simulink model "Demo1"  (R2018b)
settings: Solver=FixedStepDiscrete  StartTime=0.0  StopTime=10  FixedStep=0.0005  RelTol=1e-3  EnableMultiTasking=on
undefined symbols (not defined in the file or in its folder): ADS1, ADS2, br_opening, BRAKE, I_AN06_5V, I_AN08_5V, I_AN09_5V, I_AN10_5V, I_HALL1, I_HALL2, I_SW11_H, I_SW16_H, MnPedal_H, MnPedal_L, MxPedal_H, MxPedal_L, O_PWM1_LS0A7, O_PWM2_LS0A7, O_SW02_LS0A4, O_SW13_HS1A, O_SW14_HS1A, PUMP, th_opening
libraries: ec5744lib x93, canmsglib x14, simulink x5
(part 1 of 2)
settings Model: Creator=30855  LastModifiedBy=30855
settings OptimizationCC: DefaultParameterBehavior=Inlined  InlineInvariantSignals=on  EnhancedBackFolding=on  ExpressionFolding=off  PassReuseOutputArgsAs=Individual arguments  RollThreshold=65  StateBitsets=on  DataBitsets=on  ZeroExternalMemoryAtStartup=off  ZeroInternalMemoryAtStartup=off  EfficientFloat2IntCast=on  OptimizeBlockOrder=speed  DifferentSizesBufferReuse=on
settings DebuggingCC: InheritedTsInSrcMsg=none  ParameterTunabilityLossMsg=error
settings HardwareCC: ProdBitPerPointer=32  ProdBitPerSizeT=32  ProdBitPerPtrDiffT=32  ProdLargestAtomicInteger=Long  ProdLargestAtomicFloat=Double  ProdEndianess=BigEndian  ProdWordSize=32  ProdHWDeviceType=Freescale MPC5500
settings SFSimCC: MATLABDynamicMemAlloc=off
settings RTWCC: SystemTargetFile=ec5744.tlc  MakeCommand=make_rtw optimized_fixed_point=1  GenerateMakefile=off  TemplateMakefile=ec5744_lcc.tmf  PostCodeGenCommand=ec5744_pst_s2(buildInfo)  Description=Target for EC5744  GenerateReport=on  IncludeHyperlinkInReport=on  LaunchReport=on  GenerateTraceInfo=on  GenerateTraceReport=on  GenerateTraceReportSl=on  GenerateTraceReportSf=on  GenerateTraceReportEml=on
settings CodeAppCC: ForceParamTrailComments=on  IgnoreCustomStorageClasses=off  OperatorAnnotations=on  SimulinkDataObjDesc=on  SFDataObjDesc=on  InsertBlockDesc=on
settings STFCustomTargetCC: TargetLangStandard=C99 (ISO)  MultiwordLength=256  ModelReferenceCompliant=off  IncludeMdlTerminateFcn=off  CombineOutputUpdateFcns=on  SuppressErrorStatus=on  ERTCustomFileBanners=on  SupportContinuousTime=off  SupportNonInlinedSFcns=off  RemoveResetFunc=on  MATLABClassNameForMDSCustomization=Simulink.SoftwareTarget.ERTCustomization  SystemTargetFile=ec5744.tlc
settings ERTTargetCC: TargetLangStandard=C99 (ISO)  ModelReferenceCompliant=off  ParMdlRefBuildCompliant=off  CompOptLevelCompliant=off  ConcurrentExecutionCompliant=off  IncludeMdlTerminateFcn=off  SuppressErrorStatus=on  ModelStepFunctionPrototypeControlCompliant=off  CPPClassGenCompliant=off  UseToolchainInfoCompliant=off  GenerateASAP2=on  InlinedParameterPlacement=NonHierarchical  ERTSrcFileBannerTemplate=ec5744_code_template.cgt  ERTHdrFileBannerTemplate=ec5744_code_template.cgt  ERTDataSrcFileTemplate=ec5744_code_template.cgt  ERTDataHdrFileTemplate=ec5744_code_template.cgt  ERTCustomFileTemplate=ec5744_file_process.tlc

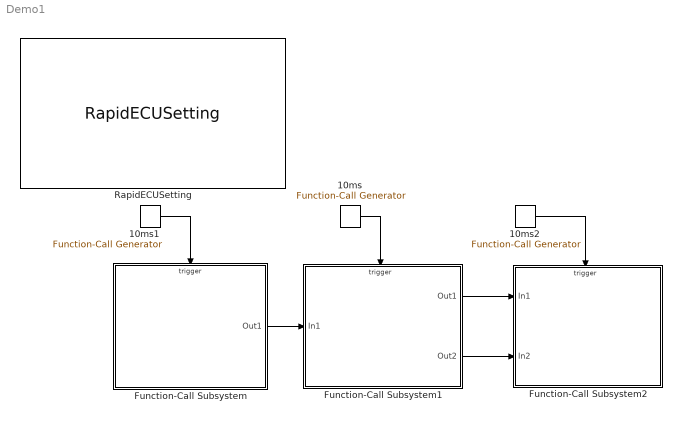
== system Demo1 ==
  10ms : simulink/Ports & Subsystems/Function-Call Generator  sample_time=0.01  numberOfIterations=1
  10ms1 : simulink/Ports & Subsystems/Function-Call Generator  sample_time=0.01  numberOfIterations=1
  10ms2 : simulink/Ports & Subsystems/Function-Call Generator  sample_time=0.01  numberOfIterations=1
  Function-Call Subsystem : Subsystem  TreatAsAtomicUnit=on
  Function-Call Subsystem1 : Subsystem  TreatAsAtomicUnit=on
  Function-Call Subsystem2 : Subsystem  TreatAsAtomicUnit=on
  RapidECUSetting : ec5744lib/RapidECU_U3/RapidECUSetting
      link override CAN: apdf=9  acmt=Extended(29-bit ID)  bpdf=9  cpdf=9  aboi=off  bcmt=Extended(29-bit ID)
      link override LIN: abrt=19200
      settings: SourceProductName=ECUCoder for MPC5744
  wires:
  10ms/1 -> Function-Call Subsystem1/Trigger
  Function-Call Subsystem/1(Out1) -> Function-Call Subsystem1/1(In1)
  Function-Call Subsystem1/1(Out1) -> Function-Call Subsystem2/1(In1)
  Function-Call Subsystem1/2(Out2) -> Function-Call Subsystem2/2(In2)
  10ms1/1 -> Function-Call Subsystem/Trigger
  10ms2/1 -> Function-Call Subsystem2/Trigger

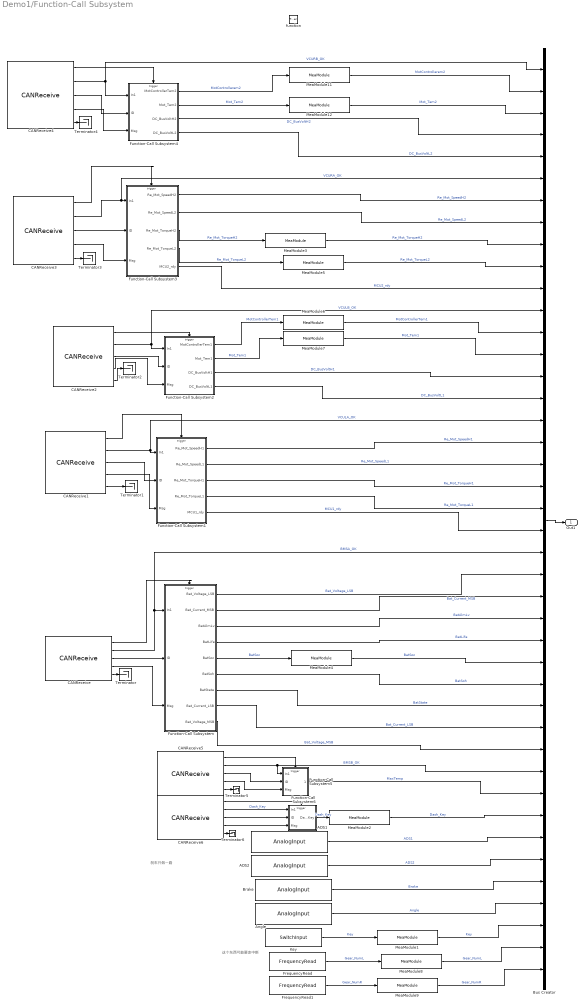
== system Demo1/Function-Call Subsystem ==
  note: 这个东西可能要走中断
  note: 刹车只做一路
  function : TriggerPort  TriggerType=function-call  VariantControl=Variant
  ADS1 : ec5744lib/RapidECU_U3/01BasicInput/AnalogInput  channel=54:I_AN08_5V  sampletime=-1
      settings: SourceProductName=ECUCoder for MPC5744
  ADS2 : ec5744lib/RapidECU_U3/01BasicInput/AnalogInput  channel=55:I_AN09_5V  sampletime=-1
      settings: SourceProductName=ECUCoder for MPC5744
  Angle : ec5744lib/RapidECU_U3/01BasicInput/AnalogInput  channel=56:I_AN10_5V  sampletime=-1
      settings: SourceProductName=ECUCoder for MPC5744
  Brake : ec5744lib/RapidECU_U3/01BasicInput/AnalogInput  channel=52:I_AN06_5V  sampletime=-1
      settings: SourceProductName=ECUCoder for MPC5744
  Bus Creator : BusCreator  Inputs=42
  CANReceive : ec5744lib/RapidECU_U3/04CANCommunication/CANReceive  canmodule=0  canbuffer=1  canmessageid=hex2dec('186040F3')  canmessagetype=Extended(29-bit ID)  datalength=8  sampletime=-1
      settings: SourceProductName=ECUCoder for MPC5744
  CANReceive1 : ec5744lib/RapidECU_U3/04CANCommunication/CANReceive  canmodule=1  canbuffer=6  canmessageid=hex2dec('CFFC6EF')  canmessagetype=Extended(29-bit ID)  datalength=8  sampletime=-1
      settings: SourceProductName=ECUCoder for MPC5744
  CANReceive2 : ec5744lib/RapidECU_U3/04CANCommunication/CANReceive  canmodule=1  canbuffer=4  canmessageid=hex2dec('CFFC7EF')  canmessagetype=Extended(29-bit ID)  datalength=8  sampletime=-1
      settings: SourceProductName=ECUCoder for MPC5744
  CANReceive3 : ec5744lib/RapidECU_U3/04CANCommunication/CANReceive  canmodule=1  canbuffer=2  canmessageid=hex2dec('CB221EF')  canmessagetype=Extended(29-bit ID)  datalength=8  sampletime=-1
      settings: SourceProductName=ECUCoder for MPC5744
  CANReceive4 : ec5744lib/RapidECU_U3/04CANCommunication/CANReceive  canmodule=1  canbuffer=0  canmessageid=hex2dec('CB321EF')  canmessagetype=Extended(29-bit ID)  datalength=8  sampletime=-1
      settings: SourceProductName=ECUCoder for MPC5744
  CANReceive5 : ec5744lib/RapidECU_U3/04CANCommunication/CANReceive  canmodule=0  canbuffer=3  canmessageid=hex2dec('186240F3')  canmessagetype=Extended(29-bit ID)  datalength=8  sampletime=-1
      settings: SourceProductName=ECUCoder for MPC5744
  CANReceive6 : ec5744lib/RapidECU_U3/04CANCommunication/CANReceive  canmodule=0  canbuffer=5  canmessageid=hex2dec('155')  canmessagetype=Extended(29-bit ID)  datalength=8  sampletime=-1
      settings: SourceProductName=ECUCoder for MPC5744
  FrequencyRead : ec5744lib/RapidECU_U3/01BasicInput/FrequencyRead  channel=37:I_HALL1  sampletime=-1
      settings: SourceProductName=ECUCoder for MPC5744
  FrequencyRead1 : ec5744lib/RapidECU_U3/01BasicInput/FrequencyRead  channel=103:I_SW16_H/I_HALL2  sampletime=-1
      settings: SourceProductName=ECUCoder for MPC5744
  Function-Call Subsystem : Subsystem  TreatAsAtomicUnit=on
  Function-Call Subsystem1 : Subsystem  TreatAsAtomicUnit=on
  Function-Call Subsystem2 : Subsystem  TreatAsAtomicUnit=on
  Function-Call Subsystem3 : Subsystem  TreatAsAtomicUnit=on
  Function-Call Subsystem4 : Subsystem  TreatAsAtomicUnit=on
  Function-Call Subsystem5 : Subsystem  TreatAsAtomicUnit=on
  Function-Call Subsystem6 : Subsystem  TreatAsAtomicUnit=on
  Key : ec5744lib/RapidECU_U3/01BasicInput/SwitchInput  channel=44:I_SW11_H  sampletime=-1
      settings: SourceProductName=ECUCoder for MPC5744
  MeaModule1 : ec5744lib/RapidECU_U3/07Calibration/MeaModule  signal=Key
      settings: SourceProductName=ECUCoder for MPC5744
  MeaModule11 : ec5744lib/RapidECU_U3/07Calibration/MeaModule  signal=MotConTem2
      settings: SourceProductName=ECUCoder for MPC5744
  MeaModule12 : ec5744lib/RapidECU_U3/07Calibration/MeaModule  signal=MotTem2
      settings: SourceProductName=ECUCoder for MPC5744
  MeaModule2 : ec5744lib/RapidECU_U3/07Calibration/MeaModule  signal=Dash_Key
      settings: SourceProductName=ECUCoder for MPC5744
  MeaModule3 : ec5744lib/RapidECU_U3/07Calibration/MeaModule  signal=Re_Mot_ToqH
      settings: SourceProductName=ECUCoder for MPC5744
  MeaModule4 : ec5744lib/RapidECU_U3/07Calibration/MeaModule  signal=BatSoc
      settings: SourceProductName=ECUCoder for MPC5744
  MeaModule5 : ec5744lib/RapidECU_U3/07Calibration/MeaModule  signal=Re_MotToqL
      settings: SourceProductName=ECUCoder for MPC5744
  MeaModule6 : ec5744lib/RapidECU_U3/07Calibration/MeaModule  signal=MotConTem1
      settings: SourceProductName=ECUCoder for MPC5744
  MeaModule7 : ec5744lib/RapidECU_U3/07Calibration/MeaModule  signal=MotTem1
      settings: SourceProductName=ECUCoder for MPC5744
  MeaModule8 : ec5744lib/RapidECU_U3/07Calibration/MeaModule  signal=HTime_L
      settings: SourceProductName=ECUCoder for MPC5744
  MeaModule9 : ec5744lib/RapidECU_U3/07Calibration/MeaModule  signal=HTime_R
      settings: SourceProductName=ECUCoder for MPC5744
  Terminator{,1..6} (7 alike) : Terminator
  Out1 : Outport
  wires:
  ADS1/1 -> Bus Creator/36  "ADS1"
  ADS2/1 -> Bus Creator/37  "ADS2"
  Brake/1 -> Bus Creator/38  "Brake"
  Angle/1 -> Bus Creator/39  "Angle"
  Bus Creator/1 -> Out1/1
  Key/1 -> MeaModule1/1  "Key"
  CANReceive/1 -> Function-Call Subsystem/Trigger
  CANReceive/2 -> Bus Creator/23, Function-Call Subsystem/1(In1)  "BMSA_OK"
  CANReceive/3 -> Function-Call Subsystem/2(ID)
  CANReceive/4 -> Function-Call Subsystem/3(Msg)
  CANReceive/5 -> Terminator/1
  Function-Call Subsystem/1(Bat_Voltage_LSB) -> Bus Creator/24  "Bat_Voltage_LSB"
  Function-Call Subsystem/2(Bat_Current_MSB) -> Bus Creator/25  "Bat_Current_MSB"
  Function-Call Subsystem/3(BatAlmLv) -> Bus Creator/26  "BatAlmLv"
  Function-Call Subsystem/4(BatLife) -> Bus Creator/27  "BatLife"
  Function-Call Subsystem/5(BatSoc) -> MeaModule4/1  "BatSoc"
  Function-Call Subsystem/6(BatSoh) -> Bus Creator/29  "BatSoh"
  Function-Call Subsystem/7(BatState) -> Bus Creator/30  "BatState"
  Function-Call Subsystem/8(Bat_Current_LSB) -> Bus Creator/31  "Bat_Current_LSB"
  FrequencyRead/1 -> MeaModule8/1  "Gear_NumL"
  CANReceive1/5 -> Terminator1/1
  CANReceive1/4 -> Function-Call Subsystem1/3(Msg)
  CANReceive1/3 -> Function-Call Subsystem1/2(ID)
  CANReceive1/2 -> Bus Creator/17, Function-Call Subsystem1/1(In1)  "VCULA_OK"
  CANReceive1/1 -> Function-Call Subsystem1/Trigger
  CANReceive2/1 -> Function-Call Subsystem2/Trigger
  CANReceive2/2 -> Function-Call Subsystem2/1(In1), Bus Creator/12  "VCULB_OK"
  CANReceive2/3 -> Function-Call Subsystem2/2(ID)
  CANReceive2/4 -> Function-Call Subsystem2/3(Msg)
  CANReceive2/5 -> Terminator2/1
  CANReceive3/5 -> Terminator3/1
  CANReceive3/4 -> Function-Call Subsystem3/3(Msg)
  CANReceive3/3 -> Function-Call Subsystem3/2(ID)
  CANReceive3/2 -> Bus Creator/6, Function-Call Subsystem3/1(In1)  "VCURA_OK"
  CANReceive3/1 -> Function-Call Subsystem3/Trigger
  CANReceive4/1 -> Function-Call Subsystem4/Trigger
  CANReceive4/2 -> Bus Creator/1, Function-Call Subsystem4/1(In1)  "VCURB_OK"
  CANReceive4/3 -> Function-Call Subsystem4/2(ID)
  CANReceive4/4 -> Function-Call Subsystem4/3(Msg)
  CANReceive4/5 -> Terminator4/1
  Function-Call Subsystem1/4(Re_Mot_TorqueL1) -> Bus Creator/21  "Re_Mot_TorqueL1"
  Function-Call Subsystem1/3(Re_Mot_TorqueH1) -> Bus Creator/20  "Re_Mot_TorqueH1"
  Function-Call Subsystem1/2(Re_Mot_SpeedL1) -> Bus Creator/19  "Re_Mot_SpeedL1"
  Function-Call Subsystem1/1(Re_Mot_SpeedH1) -> Bus Creator/18  "Re_Mot_SpeedH1"
  Function-Call Subsystem2/2(Mot_Tem1) -> MeaModule7/1  "Mot_Tem1"
  Function-Call Subsystem2/1(MotControllerTem1) -> MeaModule6/1  "MotControllerTem1"
  Function-Call Subsystem3/4(Re_Mot_TorqueL2) -> MeaModule5/1  "Re_Mot_TorqueL2"
  Function-Call Subsystem3/3(Re_Mot_TorqueH2) -> MeaModule3/1  "Re_Mot_TorqueH2"
  Function-Call Subsystem3/2(Re_Mot_SpeedL2) -> Bus Creator/8  "Re_Mot_SpeedL2"
  Function-Call Subsystem3/1(Re_Mot_SpeedH2) -> Bus Creator/7  "Re_Mot_SpeedH2"
  Function-Call Subsystem4/2(Mot_Tem2) -> MeaModule12/1  "Mot_Tem2"
  Function-Call Subsystem4/1(MotControllerTem2) -> MeaModule11/1  "MotControllerem2"
  Function-Call Subsystem/9(Bat_Voltage_MSB) -> Bus Creator/32  "Bat_Voltage_MSB"
  CANReceive5/5 -> Terminator5/1
  CANReceive5/4 -> Function-Call Subsystem5/3(Msg)
  CANReceive5/3 -> Function-Call Subsystem5/2(ID)
  CANReceive5/2 -> Bus Creator/33, Function-Call Subsystem5/1(In1)  "BMSB_OK"
  CANReceive5/1 -> Function-Call Subsystem5/Trigger
  Function-Call Subsystem5/1(MaxTemp) -> Bus Creator/34  "MaxTemp"
  FrequencyRead1/1 -> MeaModule9/1  "Gear_NumR"
  CANReceive6/1 -> Function-Call Subsystem6/Trigger
  CANReceive6/3 -> Function-Call Subsystem6/2(ID)
  CANReceive6/4 -> Function-Call Subsystem6/3(Msg)
  CANReceive6/5 -> Terminator6/1
  Function-Call Subsystem6/1(Dash_Key) -> MeaModule2/1  "Dash_Key"
  MeaModule1/1 -> Bus Creator/40  "Key"
  MeaModule3/1 -> Bus Creator/9  "Re_Mot_TorqueH2"
  MeaModule5/1 -> Bus Creator/10  "Re_Mot_TorqueL2"
  MeaModule6/1 -> Bus Creator/13  "MotControllerTem1"
  MeaModule7/1 -> Bus Creator/14  "Mot_Tem1"
  MeaModule8/1 -> Bus Creator/41  "Gear_NumL"
  MeaModule9/1 -> Bus Creator/42  "Gear_NumR"
  MeaModule11/1 -> Bus Creator/2  "MotControllerem2"
  MeaModule12/1 -> Bus Creator/3  "Mot_Tem2"
  MeaModule2/1 -> Bus Creator/35  "Dash_Key"
  CANReceive6/2 -> Function-Call Subsystem6/1(In1)  "Dash_Key"
  Function-Call Subsystem2/3(DC_BusVoltH1) -> Bus Creator/15  "DC_BusVoltH1"
  Function-Call Subsystem4/3(DC_BusVoltH2) -> Bus Creator/4  "DC_BusVoltH2"
  Function-Call Subsystem4/4(DC_BusVoltL2) -> Bus Creator/5  "DC_BusVoltL2"
  Function-Call Subsystem2/4(DC_BusVoltL1) -> Bus Creator/16  "DC_BusVoltL1"
  MeaModule4/1 -> Bus Creator/28  "BatSoc"
  Function-Call Subsystem1/5(MCU1_rdy) -> Bus Creator/22  "MCU1_rdy"
  Function-Call Subsystem3/5(MCU2_rdy) -> Bus Creator/11  "MCU2_rdy"

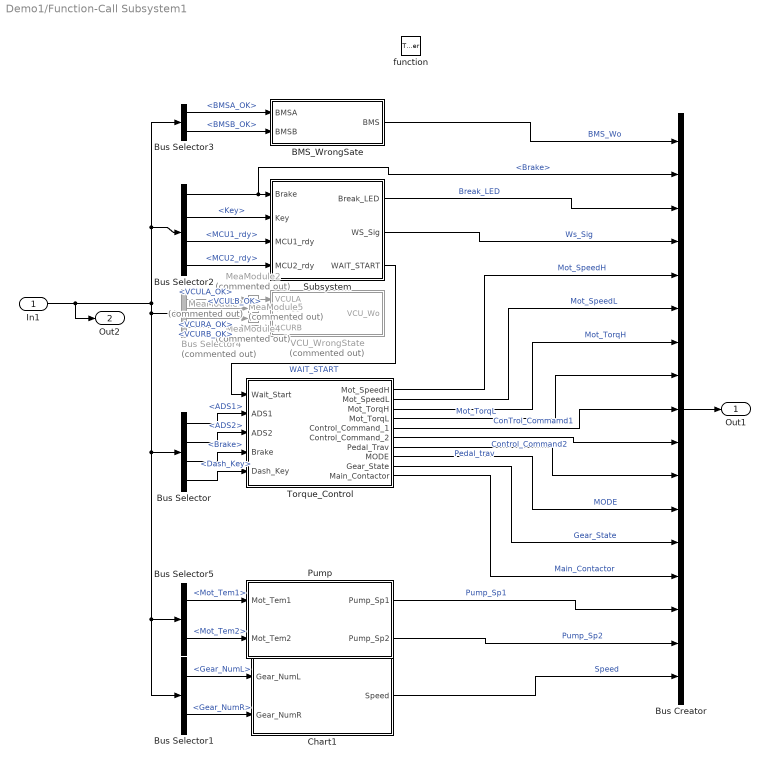
== system Demo1/Function-Call Subsystem1 ==
  In1 : Inport
  "  function" : TriggerPort  TriggerType=function-call  VariantControl=Variant
  BMS_WrongSate : Stateflow chart  TreatAsAtomicUnit=on
  Bus Creator : BusCreator  Inputs=17
  Bus Selector : BusSelector  OutputSignals=ADS1,ADS2,Brake,Dash_Key
  Bus Selector1 : BusSelector  OutputSignals=Gear_NumL,Gear_NumR
  Bus Selector2 : BusSelector  OutputSignals=Brake,Key,MCU1_rdy,MCU2_rdy
  Bus Selector3 : BusSelector  OutputSignals=BMSA_OK,BMSB_OK
  Bus Selector4 : BusSelector  Commented=on  OutputSignals=VCULA_OK,VCULB_OK,VCURA_OK,VCURB_OK
  Bus Selector5 : BusSelector  OutputSignals=Mot_Tem1,Mot_Tem2
  Chart1 : Stateflow chart  TreatAsAtomicUnit=on
  MeaModule2 : ec5744lib/RapidECU_U3/07Calibration/MeaModule  Commented=on  signal=VCULA
      settings: SourceProductName=ECUCoder for MPC5744
  MeaModule3 : ec5744lib/RapidECU_U3/07Calibration/MeaModule  Commented=on  signal=VCUlb
      settings: SourceProductName=ECUCoder for MPC5744
  MeaModule4 : ec5744lib/RapidECU_U3/07Calibration/MeaModule  Commented=on  signal=VCUra
      settings: SourceProductName=ECUCoder for MPC5744
  MeaModule5 : ec5744lib/RapidECU_U3/07Calibration/MeaModule  Commented=on  signal=VCUrb
      settings: SourceProductName=ECUCoder for MPC5744
  Pump : Subsystem
  Subsystem : Subsystem
  Torque_Control : Subsystem
  VCU_WrongState : Stateflow chart  Commented=on  TreatAsAtomicUnit=on
  Out1 : Outport
  Out2 : Outport  Port=2
  wires:
  Bus Selector/1 -> Torque_Control/2(ADS1)  "<ADS1>"
  Bus Selector/2 -> Torque_Control/3(ADS2)  "<ADS2>"
  Torque_Control/1(Mot_SpeedH) -> Bus Creator/5  "Mot_SpeedH"
  Torque_Control/2(Mot_SpeedL) -> Bus Creator/6  "Mot_SpeedL"
  Torque_Control/3(Mot_TorqH) -> Bus Creator/7  "Mot_TorqH"
  Torque_Control/4(Mot_TorqL) -> Bus Creator/8  "Mot_TorqL"
  Bus Creator/1 -> Out1/1
  Bus Selector2/2 -> Subsystem/2(Key)  "<Key>"
  Subsystem/3(WAIT_START) -> Torque_Control/1(Wait_Start)  "WAIT_START"
  BMS_WrongSate/1(BMS) -> Bus Creator/1  "BMS_Wo"
  Torque_Control/5("Control_Command_1 ") -> Bus Creator/9  "ConTrol_Commamd1"
  Torque_Control/6(Control_Command_2) -> Bus Creator/10  "Control_Command2"
  Bus Selector2/1 -> Bus Creator/2, Subsystem/1(Brake)  "<Brake>"
  Torque_Control/7(Pedal_Trav) -> Bus Creator/11  "Pedal_trav"
  Bus Selector/4 -> Torque_Control/5("Dash_Key ")  "<Dash_Key>"
  Bus Selector5/1 -> Pump/1(Mot_Tem1)  "<Mot_Tem1>"
  Bus Selector5/2 -> Pump/2(Mot_Tem2)  "<Mot_Tem2>"
  Pump/1(Pump_Sp1) -> Bus Creator/15  "Pump_Sp1"
  Pump/2(Pump_Sp2) -> Bus Creator/16  "Pump_Sp2"
  Subsystem/1(Break_LED) -> Bus Creator/3  "Break_LED"
  Bus Selector/3 -> Torque_Control/4("Brake ")  "<Brake>"
  Bus Selector3/1 -> BMS_WrongSate/1(BMSA)  "<BMSA_OK>"
  Bus Selector3/2 -> BMS_WrongSate/2(BMSB)  "<BMSB_OK>"
  Bus Selector4/1 -> MeaModule2/1  "<VCULA_OK>"
  Bus Selector4/2 -> MeaModule3/1  "<VCULB_OK>"
  Bus Selector4/3 -> MeaModule4/1  "<VCURA_OK>"
  Bus Selector4/4 -> MeaModule5/1  "<VCURB_OK>"
  MeaModule2/1 -> VCU_WrongState/1(VCULA)
  MeaModule3/1 -> VCU_WrongState/2(VCULB)
  MeaModule4/1 -> VCU_WrongState/3(VCURA)
  MeaModule5/1 -> VCU_WrongState/4(VCURB)
  Bus Selector1/2 -> Chart1/2(Gear_NumR)  "<Gear_NumR>"
  Bus Selector1/1 -> Chart1/1(Gear_NumL)  "<Gear_NumL>"
  In1/1 -> Out2/1, Bus Selector4/1, Bus Selector1/1, Bus Selector5/1, Bus Selector/1, Bus Selector3/1, Bus Selector2/1
  Chart1/1(Speed) -> Bus Creator/17  "Speed"
  Torque_Control/8(MODE) -> Bus Creator/12  "MODE"
  Subsystem/2(WS_Sig) -> Bus Creator/4  "Ws_Sig"
  Torque_Control/9("Gear_State ") -> Bus Creator/13  "Gear_State"
  Torque_Control/10(Main_Contactor) -> Bus Creator/14  "Main_Contactor"
  Bus Selector2/3 -> Subsystem/3(MCU1_rdy)  "<MCU1_rdy>"
  Bus Selector2/4 -> Subsystem/4(MCU2_rdy)  "<MCU2_rdy>"

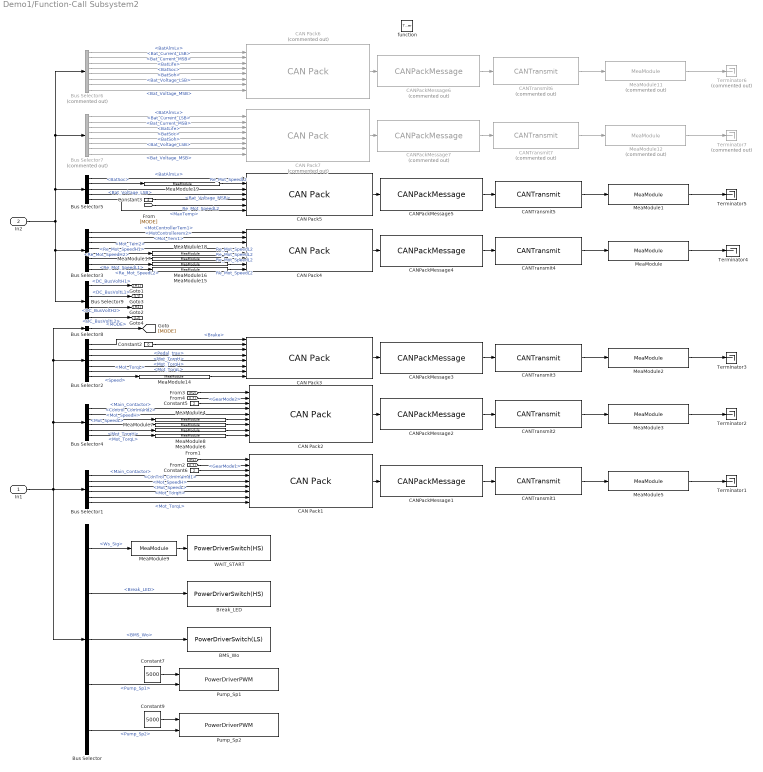
== system Demo1/Function-Call Subsystem2 ==
  In1 : Inport
  In2 : Inport  Port=2
  function : TriggerPort  TriggerType=function-call  VariantControl=Variant
  BMS_Wo : ec5744lib/RapidECU_U3/02PowerDriverSwitch/PowerDriverSwitch(LS)  channel=59:O_SW02_LS0A4  sampletime=-1
      settings: SourceProductName=ECUCoder for MPC5744
  Break_LED : ec5744lib/RapidECU_U3/02PowerDriverSwitch/PowerDriverSwitch(HS)  channel=115:O_SW13_HS1A  sampletime=-1
      settings: SourceProductName=ECUCoder for MPC5744
  Bus Selector : BusSelector  OutputSignals=Ws_Sig,Break_LED,BMS_Wo,Pump_Sp1,Pump_Sp2
  Bus Selector1 : BusSelector  OutputSignals=Main_Contactor,ConTrol_Commamd1,Mot_SpeedH,Mot_SpeedL,Mot_TorqH,Mot_TorqL
  Bus Selector2 : BusSelector  OutputSignals=Brake,Pedal_trav,Mot_TorqH,Mot_TorqH,Mot_TorqL,Mot_TorqL,Speed
  Bus Selector3 : BusSelector  OutputSignals=MotControllerTem1,MotControllerem2,Mot_Tem1,Mot_Tem2,Re_Mot_SpeedH1,Re_Mot_SpeedH2,Re_Mot_SpeedL1,Re_Mot_SpeedL2
  Bus Selector4 : BusSelector  OutputSignals=Main_Contactor,Control_Command2,Mot_SpeedH,Mot_SpeedL,Mot_TorqH,Mot_TorqL
  Bus Selector5 : BusSelector  OutputSignals=BatAlmLv,BatSoc,Bat_Voltage_LSB,Bat_Voltage_MSB,MaxTemp
  Bus Selector6 : BusSelector  Commented=on  OutputSignals=BatAlmLv,Bat_Current_LSB,Bat_Current_MSB,BatLife,BatSoc,BatSoh,Bat_Voltage_LSB,Bat_Voltage_MSB
  Bus Selector7 : BusSelector  Commented=on  OutputSignals=BatAlmLv,Bat_Current_LSB,Bat_Current_MSB,BatLife,BatSoc,BatSoh,Bat_Voltage_LSB,Bat_Voltage_MSB
  Bus Selector8 : BusSelector  OutputSignals=MODE
  Bus Selector9 : BusSelector  OutputSignals=DC_BusVoltH1,DC_BusVoltL1,DC_BusVoltH2,DC_BusVoltL2
  CAN Pack1 : canmsglib/CAN Pack  CANdbFile=E:\project\DBC_file\MotControl.dbc  MsgList=VCUtoMUC1  MsgName=VCUtoMUC1  MsgIDType=Extended (29-bit identifier)  MsgIdentifier=146927393  MsgLength=8  SignalInfo=DC_Bus_VoltageH1$48$8$1$2$1$0$1$0$0$255$#DC_Bus_VoltageL1$56$8$1$2$1$0$1$0$0$255$#GearState1$40$2$1$2$1$0$1$0$0$3$#Main_contactor1$43$1$1$2$1$0$1$0$0$1$#Tr_ControlMode_Command1$32$8$1$2$1$0$1$0$0$255$#Tr_Mot_SpeedH1$8$8$1$2$1$0$1$0$0$255$#Tr_Mot_SpeedL1$0$8$1$2$1$0$1$0$0$255$#Tr_Mot_TorqH1$24$8$1$2$1$0$1$0$0$255$#Tr_Mot_TorqL1$16$8$1$2$1$0$1$0$0$255$#  NSignals=9  StartBits=str2num('[int32(48);int32(56);int32(40);int32(43);int32(32);int32(8);int32(0);int32(24);int32(16)]')  SignalSizes=str2num('[int32(8);int32(8);int32(2);int32(1);int32(8);int32(8);int32(8);int32(8);int32(8)]')  ByteOrders=str2num('[int32(1);int32(1);int32(1);int32(1);int32(1);int32(1);int32(1);int32(1);int32(1)]')  DataTypes=str2num('[int32(2);int32(2);int32(2);int32(2);int32(2);int32(2);int32(2);int32(2);int32(2)]')  MultiplexTypes=str2num('[int32(1);int32(1);int32(1);int32(1);int32(1);int32(1);int32(1);int32(1);int32(1)]')  MultiplexValues=str2num('[double(0);double(0);double(0);double(0);double(0);double(0);double(0);double(0);double(0)]')  Factors=str2num('[double(1);double(1);double(1);double(1);double(1);double(1);double(1);double(1);double(1)]')  Offsets=str2num('[double(0);double(0);double(0);double(0);double(0);double(0);double(0);double(0);double(0)]')  Minimums=str2num('[double(0);double(0);double(0);double(0);double(0);double(0);double(0);double(0);double(0)]')  Maximums=str2num('[double(255);double(255);double(3);double(1);double(255);double(255);double(255);double(255);double(255)]')  Remote=off  ApplyMinMax=off  BusOutput=off
      settings: SourceProductName=Simulink Real-Time  SourceProductBaseCode=XP  DataFormat=CANdb specified signals
  CAN Pack2 : canmsglib/CAN Pack  CANdbFile=E:\project\DBC_file\MotControl.dbc  MsgList=VCUtoMCU2  MsgName=VCUtoMCU2  MsgIDType=Extended (29-bit identifier)  MsgIdentifier=145878817  MsgLength=8  SignalInfo=DC_Bus_VoltageH2$48$8$1$2$1$0$1$0$0$255$#DC_Bus_VoltrageL2$56$8$1$2$1$0$1$0$0$255$#GearState2$40$2$1$2$1$0$1$0$0$3$#Main_contactor2$43$1$1$2$1$0$1$0$0$1$#Tr_ControlMode_Command2$32$8$1$2$1$0$1$0$0$255$#Tr_Mot_SpeedH2$8$8$1$2$1$0$1$0$0$255$#Tr_Mot_SpeedL2$0$8$1$2$1$0$1$0$0$255$#Tr_Mot_TorqH2$24$8$1$2$1$0$1$0$0$255$#Tr_Mot_TorqL2$16$8$1$2$1$0$1$0$0$255$#  NSignals=9  StartBits=str2num('[int32(48);int32(56);int32(40);int32(43);int32(32);int32(8);int32(0);int32(24);int32(16)]')  SignalSizes=str2num('[int32(8);int32(8);int32(2);int32(1);int32(8);int32(8);int32(8);int32(8);int32(8)]')  ByteOrders=str2num('[int32(1);int32(1);int32(1);int32(1);int32(1);int32(1);int32(1);int32(1);int32(1)]')  DataTypes=str2num('[int32(2);int32(2);int32(2);int32(2);int32(2);int32(2);int32(2);int32(2);int32(2)]')  MultiplexTypes=str2num('[int32(1);int32(1);int32(1);int32(1);int32(1);int32(1);int32(1);int32(1);int32(1)]')  MultiplexValues=str2num('[double(0);double(0);double(0);double(0);double(0);double(0);double(0);double(0);double(0)]')  Factors=str2num('[double(1);double(1);double(1);double(1);double(1);double(1);double(1);double(1);double(1)]')  Offsets=str2num('[double(0);double(0);double(0);double(0);double(0);double(0);double(0);double(0);double(0)]')  Minimums=str2num('[double(0);double(0);double(0);double(0);double(0);double(0);double(0);double(0);double(0)]')  Maximums=str2num('[double(255);double(255);double(3);double(1);double(255);double(255);double(255);double(255);double(255)]')  Remote=off  ApplyMinMax=off  BusOutput=off
      settings: SourceProductName=Simulink Real-Time  SourceProductBaseCode=XP  DataFormat=CANdb specified signals
  CAN Pack3 : canmsglib/CAN Pack  CANdbFile=E:\project\DBC_file\MotControl.dbc  MsgList=VCUtoDash1  MsgName=VCUtoDash1  MsgIDType=Extended (29-bit identifier)  MsgIdentifier=529  MsgLength=8  SignalInfo=Brake_Val$16$8$1$2$1$0$1$0$0$255$#Distance$24$8$1$2$1$0$1$0$0$255$#Ped_Trav$8$8$1$2$1$0$1$0$0$255$#Re_Mot_TorqueH1$40$8$1$2$1$0$1$0$0$255$#Re_Mot_TorqueH2$56$8$1$2$1$0$1$0$0$255$#Re_Mot_TorqueL1$32$8$1$2$1$0$1$0$0$255$#Re_Mot_TorqueL2$48$8$1$2$1$0$1$0$0$255$#Veh_Sp$0$8$1$2$1$0$1$0$0$255$#  NSignals=8  StartBits=str2num('[int32(16);int32(24);int32(8);int32(40);int32(56);int32(32);int32(48);int32(0)]')  SignalSizes=str2num('[int32(8);int32(8);int32(8);int32(8);int32(8);int32(8);int32(8);int32(8)]')  ByteOrders=str2num('[int32(1);int32(1);int32(1);int32(1);int32(1);int32(1);int32(1);int32(1)]')  DataTypes=str2num('[int32(2);int32(2);int32(2);int32(2);int32(2);int32(2);int32(2);int32(2)]')  MultiplexTypes=str2num('[int32(1);int32(1);int32(1);int32(1);int32(1);int32(1);int32(1);int32(1)]')  MultiplexValues=str2num('[double(0);double(0);double(0);double(0);double(0);double(0);double(0);double(0)]')  Factors=str2num('[double(1);double(1);double(1);double(1);double(1);double(1);double(1);double(1)]')  Offsets=str2num('[double(0);double(0);double(0);double(0);double(0);double(0);double(0);double(0)]')  Minimums=str2num('[double(0);double(0);double(0);double(0);double(0);double(0);double(0);double(0)]')  Maximums=str2num('[double(255);double(255);double(255);double(255);double(255);double(255);double(255);double(255)]')  Remote=off  ApplyMinMax=off  BusOutput=off
      settings: SourceProductName=Simulink Real-Time  SourceProductBaseCode=XP  DataFormat=CANdb specified signals
  CAN Pack4 : canmsglib/CAN Pack  CANdbFile=E:\project\DBC_file\MotControl.dbc  MsgList=VCUtoDash2  MsgName=VCUtoDash2  MsgIDType=Extended (29-bit identifier)  MsgIdentifier=530  MsgLength=8  SignalInfo=MotControllerTem1$24$8$1$2$1$0$1$0$0$255$#MotControllerTem2$56$8$1$2$1$0$1$0$0$255$#Mot_Tem1$16$8$1$2$1$0$1$0$0$255$#Mot_Tem2$48$8$1$2$1$0$1$0$0$255$#Re_Mot_SpeedH1$8$8$1$2$1$0$1$0$0$255$#Re_Mot_SpeedH2$40$8$1$2$1$0$1$0$0$255$#Re_Mot_SpeedL1$0$8$1$2$1$0$1$0$0$255$#Re_Mot_SpeedL2$32$8$1$2$1$0$1$0$0$255$#  NSignals=8  StartBits=str2num('[int32(24);int32(56);int32(16);int32(48);int32(8);int32(40);int32(0);int32(32)]')  SignalSizes=str2num('[int32(8);int32(8);int32(8);int32(8);int32(8);int32(8);int32(8);int32(8)]')  ByteOrders=str2num('[int32(1);int32(1);int32(1);int32(1);int32(1);int32(1);int32(1);int32(1)]')  DataTypes=str2num('[int32(2);int32(2);int32(2);int32(2);int32(2);int32(2);int32(2);int32(2)]')  MultiplexTypes=str2num('[int32(1);int32(1);int32(1);int32(1);int32(1);int32(1);int32(1);int32(1)]')  MultiplexValues=str2num('[double(0);double(0);double(0);double(0);double(0);double(0);double(0);double(0)]')  Factors=str2num('[double(1);double(1);double(1);double(1);double(1);double(1);double(1);double(1)]')  Offsets=str2num('[double(0);double(0);double(0);double(0);double(0);double(0);double(0);double(0)]')  Minimums=str2num('[double(0);double(0);double(0);double(0);double(0);double(0);double(0);double(0)]')  Maximums=str2num('[double(255);double(255);double(255);double(255);double(255);double(255);double(255);double(255)]')  Remote=off  ApplyMinMax=off  BusOutput=off
      settings: SourceProductName=Simulink Real-Time  SourceProductBaseCode=XP  DataFormat=CANdb specified signals
  CAN Pack5 : canmsglib/CAN Pack  CANdbFile=E:\project\DBC_file\MotControl.dbc  MsgList=VCUtoDash3  MsgName=VCUtoDash3  MsgIDType=Extended (29-bit identifier)  MsgIdentifier=531  MsgLength=8  SignalInfo=BatAlmLv$0$4$1$2$1$0$1$0$0$15$#BatSoc$16$8$1$2$1$0$1$0$0$255$#BatVoltage_LSB$24$8$1$2$1$0$1$0$0$255$#BatVoltage_MSB$32$8$1$2$1$0$1$0$0$255$#ControlMode_Command1$48$8$1$2$1$0$1$0$0$255$#GearState$40$2$1$2$1$0$1$0$0$3$#MaxTemp$8$8$1$2$1$0$1$0$0$255$#  NSignals=7  StartBits=str2num('[int32(0);int32(16);int32(24);int32(32);int32(48);int32(40);int32(8)]')  SignalSizes=str2num('[int32(4);int32(8);int32(8);int32(8);int32(8);int32(2);int32(8)]')  ByteOrders=str2num('[int32(1);int32(1);int32(1);int32(1);int32(1);int32(1);int32(1)]')  DataTypes=str2num('[int32(2);int32(2);int32(2);int32(2);int32(2);int32(2);int32(2)]')  MultiplexTypes=str2num('[int32(1);int32(1);int32(1);int32(1);int32(1);int32(1);int32(1)]')  MultiplexValues=str2num('[double(0);double(0);double(0);double(0);double(0);double(0);double(0)]')  Factors=str2num('[double(1);double(1);double(1);double(1);double(1);double(1);double(1)]')  Offsets=str2num('[double(0);double(0);double(0);double(0);double(0);double(0);double(0)]')  Minimums=str2num('[double(0);double(0);double(0);double(0);double(0);double(0);double(0)]')  Maximums=str2num('[double(15);double(255);double(255);double(255);double(255);double(3);double(255)]')  Remote=off  ApplyMinMax=off  BusOutput=off
      settings: SourceProductName=Simulink Real-Time  SourceProductBaseCode=XP  DataFormat=CANdb specified signals
  CAN Pack6 : canmsglib/CAN Pack  Commented=on  CANdbFile=E:\project\DBC_file\MotControl.dbc  MsgList=VCU_Com1  MsgName=VCU_Com1  MsgIDType=Extended (29-bit identifier)  MsgIdentifier=140525809  MsgLength=8  SignalInfo=BatAlmLv$32$4$1$2$1$0$1$0$0$15$#BatCurrent_LSB$0$8$1$2$1$0$1$0$0$255$#BatCurrent_MSB$8$8$1$2$1$0$1$0$0$255$#BatLife$16$8$1$2$1$0$1$0$0$255$#BatSoc$24$8$1$2$1$0$1$0$0$255$#BatSoh$40$8$1$2$1$0$1$0$0$255$#BatVoltage_LSB$48$8$1$2$1$0$1$0$0$255$#BatVoltage_MSB$56$8$1$2$1$0$1$0$0$255$#  NSignals=8  StartBits=str2num('[int32(32);int32(0);int32(8);int32(16);int32(24);int32(40);int32(48);int32(56)]')  SignalSizes=str2num('[int32(4);int32(8);int32(8);int32(8);int32(8);int32(8);int32(8);int32(8)]')  ByteOrders=str2num('[int32(1);int32(1);int32(1);int32(1);int32(1);int32(1);int32(1);int32(1)]')  DataTypes=str2num('[int32(2);int32(2);int32(2);int32(2);int32(2);int32(2);int32(2);int32(2)]')  MultiplexTypes=str2num('[int32(1);int32(1);int32(1);int32(1);int32(1);int32(1);int32(1);int32(1)]')  MultiplexValues=str2num('[double(0);double(0);double(0);double(0);double(0);double(0);double(0);double(0)]')  Factors=str2num('[double(1);double(1);double(1);double(1);double(1);double(1);double(1);double(1)]')  Offsets=str2num('[double(0);double(0);double(0);double(0);double(0);double(0);double(0);double(0)]')  Minimums=str2num('[double(0);double(0);double(0);double(0);double(0);double(0);double(0);double(0)]')  Maximums=str2num('[double(15);double(255);double(255);double(255);double(255);double(255);double(255);double(255)]')  Remote=off  ApplyMinMax=off  BusOutput=off
      settings: SourceProductName=Simulink Real-Time  SourceProductBaseCode=XP  DataFormat=CANdb specified signals
  CAN Pack7 : canmsglib/CAN Pack  Commented=on  CANdbFile=E:\project\DBC_file\MotControl.dbc  MsgList=VCU_Com2  MsgName=VCU_Com2  MsgIDType=Extended (29-bit identifier)  MsgIdentifier=140525810  MsgLength=8  SignalInfo=BatAlmLv$0$4$1$2$1$0$1$0$0$15$#BatCurrent_LSB$8$8$1$2$1$0$1$0$0$255$#BatCurrent_MSB$16$8$1$2$1$0$1$0$0$255$#BatLife$24$8$1$2$1$0$1$0$0$255$#BatSoc$32$8$1$2$1$0$1$0$0$255$#BatSoh$40$8$1$2$1$0$1$0$0$255$#BatVoltage_LSB$48$8$1$2$1$0$1$0$0$255$#BatVoltage_MSB$56$8$1$2$1$0$1$0$0$255$#  NSignals=8  StartBits=str2num('[int32(0);int32(8);int32(16);int32(24);int32(32);int32(40);int32(48);int32(56)]')  SignalSizes=str2num('[int32(4);int32(8);int32(8);int32(8);int32(8);int32(8);int32(8);int32(8)]')  ByteOrders=str2num('[int32(1);int32(1);int32(1);int32(1);int32(1);int32(1);int32(1);int32(1)]')  DataTypes=str2num('[int32(2);int32(2);int32(2);int32(2);int32(2);int32(2);int32(2);int32(2)]')  MultiplexTypes=str2num('[int32(1);int32(1);int32(1);int32(1);int32(1);int32(1);int32(1);int32(1)]')  MultiplexValues=str2num('[double(0);double(0);double(0);double(0);double(0);double(0);double(0);double(0)]')  Factors=str2num('[double(1);double(1);double(1);double(1);double(1);double(1);double(1);double(1)]')  Offsets=str2num('[double(0);double(0);double(0);double(0);double(0);double(0);double(0);double(0)]')  Minimums=str2num('[double(0);double(0);double(0);double(0);double(0);double(0);double(0);double(0)]')  Maximums=str2num('[double(15);double(255);double(255);double(255);double(255);double(255);double(255);double(255)]')  Remote=off  ApplyMinMax=off  BusOutput=off
      settings: SourceProductName=Simulink Real-Time  SourceProductBaseCode=XP  DataFormat=CANdb specified signals
  CANPackMessage{1..5} (5 alike) : ec5744lib/RapidECU_U3/04CANCommunication/CANPackMessage  datalength=8  sampletime=-1
      settings: SourceProductName=ECUCoder for MPC5744
  CANPackMessage6 : ec5744lib/RapidECU_U3/04CANCommunication/CANPackMessage  Commented=on  datalength=8  sampletime=-1
      settings: SourceProductName=ECUCoder for MPC5744
  CANPackMessage7 : ec5744lib/RapidECU_U3/04CANCommunication/CANPackMessage  Commented=on  datalength=8  sampletime=-1
      settings: SourceProductName=ECUCoder for MPC5744
  CANTransmit1 : ec5744lib/RapidECU_U3/04CANCommunication/CANTransmit  canmodule=1  canbuffer=12  canmessageid=hex2dec('8C1EF21')  canmessagetype=Extended(29-bit ID)  datalength=8  sampletime=-1
      settings: SourceProductName=ECUCoder for MPC5744
  CANTransmit2 : ec5744lib/RapidECU_U3/04CANCommunication/CANTransmit  canmodule=1  canbuffer=10  canmessageid=hex2dec('8B1EF21')  canmessagetype=Extended(29-bit ID)  datalength=8  sampletime=-1
      settings: SourceProductName=ECUCoder for MPC5744
  CANTransmit3 : ec5744lib/RapidECU_U3/04CANCommunication/CANTransmit  canmodule=0  canbuffer=12  canmessageid=hex2dec('211')  canmessagetype=Extended(29-bit ID)  datalength=8  sampletime=-1
      settings: SourceProductName=ECUCoder for MPC5744
  CANTransmit4 : ec5744lib/RapidECU_U3/04CANCommunication/CANTransmit  canmodule=0  canbuffer=11  canmessageid=hex2dec('212')  canmessagetype=Extended(29-bit ID)  datalength=8  sampletime=-1
      settings: SourceProductName=ECUCoder for MPC5744
  CANTransmit5 : ec5744lib/RapidECU_U3/04CANCommunication/CANTransmit  canmodule=0  canbuffer=10  canmessageid=hex2dec('213')  canmessagetype=Extended(29-bit ID)  datalength=8  sampletime=-1
      settings: SourceProductName=ECUCoder for MPC5744
  CANTransmit6 : ec5744lib/RapidECU_U3/04CANCommunication/CANTransmit  Commented=on  canmodule=0  canbuffer=8  canmessageid=hex2dec('251')  canmessagetype=Extended(29-bit ID)  datalength=8  sampletime=-1
      settings: SourceProductName=ECUCoder for MPC5744
  CANTransmit7 : ec5744lib/RapidECU_U3/04CANCommunication/CANTransmit  Commented=on  canmodule=0  canbuffer=9  canmessageid=hex2dec('252')  canmessagetype=Extended(29-bit ID)  datalength=8  sampletime=-1
      settings: SourceProductName=ECUCoder for MPC5744
  Constant2 : Constant  Value=0
  Constant3 : Constant  Value=2
  Constant5 : Constant  Value=2
  Constant6 : Constant  Value=2
  Constant7 : Constant  Value=5000  OutDataTypeStr=uint16
  Constant9 : Constant  Value=5000  OutDataTypeStr=uint16
  MeaModule : ec5744lib/RapidECU_U3/07Calibration/MeaModule  signal=Dash2
      settings: SourceProductName=ECUCoder for MPC5744
  MeaModule1 : ec5744lib/RapidECU_U3/07Calibration/MeaModule  signal=Dash3
      settings: SourceProductName=ECUCoder for MPC5744
  MeaModule11 : ec5744lib/RapidECU_U3/07Calibration/MeaModule  Commented=on  signal=VCU_Com1
      settings: SourceProductName=ECUCoder for MPC5744
  MeaModule12 : ec5744lib/RapidECU_U3/07Calibration/MeaModule  Commented=on  signal=VCU_Com2
      settings: SourceProductName=ECUCoder for MPC5744
  MeaModule14 : ec5744lib/RapidECU_U3/07Calibration/MeaModule  signal=Vh_Speed
      settings: SourceProductName=ECUCoder for MPC5744
  MeaModule15 : ec5744lib/RapidECU_U3/07Calibration/MeaModule  signal=Re_Mot_SpeedL2
      settings: SourceProductName=ECUCoder for MPC5744
  MeaModule16 : ec5744lib/RapidECU_U3/07Calibration/MeaModule  signal=Re_Mot_SpeedL1
      settings: SourceProductName=ECUCoder for MPC5744
  MeaModule17 : ec5744lib/RapidECU_U3/07Calibration/MeaModule  signal=Re_Mot_SpeedH2
      settings: SourceProductName=ECUCoder for MPC5744
  MeaModule18 : ec5744lib/RapidECU_U3/07Calibration/MeaModule  signal=Re_Mot_SpeedH1
      settings: SourceProductName=ECUCoder for MPC5744
  MeaModule19 : ec5744lib/RapidECU_U3/07Calibration/MeaModule  signal=BatSOC
      settings: SourceProductName=ECUCoder for MPC5744
  MeaModule2 : ec5744lib/RapidECU_U3/07Calibration/MeaModule  signal=Dash1
      settings: SourceProductName=ECUCoder for MPC5744
  MeaModule3 : ec5744lib/RapidECU_U3/07Calibration/MeaModule  signal=VCUtoMCU2
      settings: SourceProductName=ECUCoder for MPC5744
  MeaModule4 : ec5744lib/RapidECU_U3/07Calibration/MeaModule  signal=SpeedH
      settings: SourceProductName=ECUCoder for MPC5744
  MeaModule5 : ec5744lib/RapidECU_U3/07Calibration/MeaModule  signal=VCUtoMCU
      settings: SourceProductName=ECUCoder for MPC5744
  MeaModule6 : ec5744lib/RapidECU_U3/07Calibration/MeaModule  signal=TorqL
      settings: SourceProductName=ECUCoder for MPC5744
  MeaModule7 : ec5744lib/RapidECU_U3/07Calibration/MeaModule  signal=SpeedL
      settings: SourceProductName=ECUCoder for MPC5744
  MeaModule8 : ec5744lib/RapidECU_U3/07Calibration/MeaModule  signal=TorqH
      settings: SourceProductName=ECUCoder for MPC5744
  MeaModule9 : ec5744lib/RapidECU_U3/07Calibration/MeaModule  signal=Ws_Sig
      settings: SourceProductName=ECUCoder for MPC5744
  Pump_Sp1 : ec5744lib/RapidECU_U3/03PowerDriverPWM/PowerDriverPWM  channel=60:O_PWM1_LS0A7  sampletime=-1
      settings: SourceProductName=ECUCoder for MPC5744
  Pump_Sp2 : ec5744lib/RapidECU_U3/03PowerDriverPWM/PowerDriverPWM  channel=90:O_PWM2_LS0A7  sampletime=-1
      settings: SourceProductName=ECUCoder for MPC5744
  Terminator{1..5} (5 alike) : Terminator
  Terminator6 : Terminator  Commented=on
  Terminator7 : Terminator  Commented=on
  WAIT_START : ec5744lib/RapidECU_U3/02PowerDriverSwitch/PowerDriverSwitch(HS)  channel=117:O_SW14_HS1A  sampletime=-1
      settings: SourceProductName=ECUCoder for MPC5744
  wires:
  CANPackMessage1/1 -> CANTransmit1/1
  CANTransmit1/1 -> MeaModule5/1
  Bus Selector/1 -> MeaModule9/1  "<Ws_Sig>"
  CANTransmit2/1 -> MeaModule3/1
  CANPackMessage2/1 -> CANTransmit2/1
  Bus Selector4/5 -> MeaModule8/1  "<Mot_TorqH>"
  Bus Selector4/6 -> MeaModule6/1  "<Mot_TorqL>"
  Bus Selector4/3 -> MeaModule4/1  "<Mot_SpeedH>"
  Bus Selector4/4 -> MeaModule7/1  "<Mot_SpeedL>"
  Constant5/1 -> CAN Pack2/3  "<GearMode2>"
  Constant6/1 -> CAN Pack1/3  "<GearMode1>"
  Bus Selector1/2 -> CAN Pack1/5  "<ConTrol_Commamd1>"
  Bus Selector1/4 -> CAN Pack1/7  "<Mot_SpeedL>"
  Bus Selector1/3 -> CAN Pack1/6  "<Mot_SpeedH>"
  Bus Selector1/6 -> CAN Pack1/9  "<Mot_TorqL>"
  Bus Selector1/5 -> CAN Pack1/8  "<Mot_TorqH>"
  CAN Pack3/1 -> CANPackMessage3/1
  CAN Pack4/1 -> CANPackMessage4/1
  CAN Pack5/1 -> CANPackMessage5/1
  CANPackMessage3/1 -> CANTransmit3/1
  CANPackMessage4/1 -> CANTransmit4/1
  CANPackMessage5/1 -> CANTransmit5/1
  CANTransmit3/1 -> MeaModule2/1
  CANTransmit4/1 -> MeaModule/1
  CANTransmit5/1 -> MeaModule1/1
  In1/1 -> Bus Selector/1, Bus Selector1/1, Bus Selector8/1, Bus Selector2/1, Bus Selector4/1
  Constant2/1 -> CAN Pack3/2
  Bus Selector2/2 -> CAN Pack3/3  "<Pedal_trav>"
  Bus Selector2/3 -> CAN Pack3/4  "<Mot_TorqH>"
  Bus Selector2/4 -> CAN Pack3/5  "<Mot_TorqH>"
  Bus Selector2/5 -> CAN Pack3/6  "<Mot_TorqL>"
  Bus Selector2/6 -> CAN Pack3/7  "<Mot_TorqL>"
  In2/1 -> Bus Selector9/1, Bus Selector3/1, Bus Selector7/1, Bus Selector6/1, Bus Selector5/1
  Bus Selector5/1 -> CAN Pack5/1  "<BatAlmLv>"
  Bus Selector5/3 -> CAN Pack5/3  "<Bat_Voltage_LSB>"
  Bus Selector5/2 -> MeaModule19/1  "<BatSoc>"
  Bus Selector5/4 -> CAN Pack5/4  "<Bat_Voltage_MSB>"
  Bus Selector5/5 -> CAN Pack5/7  "<MaxTemp>"
  Constant3/1 -> CAN Pack5/5
  MeaModule/1 -> Terminator4/1
  MeaModule1/1 -> Terminator5/1
  MeaModule2/1 -> Terminator3/1
  MeaModule3/1 -> Terminator2/1
  MeaModule5/1 -> Terminator1/1
  Bus Selector/4 -> Pump_Sp1/2  "<Pump_Sp1>"
  Bus Selector/5 -> Pump_Sp2/2  "<Pump_Sp2>"
  Bus Selector/2 -> Break_LED/1  "<Break_LED>"
  Constant7/1 -> Pump_Sp1/1
  Constant9/1 -> Pump_Sp2/1
  Bus Selector4/2 -> CAN Pack2/5  "<Control_Command2>"
  MeaModule4/1 -> CAN Pack2/6
  MeaModule7/1 -> CAN Pack2/7
  MeaModule8/1 -> CAN Pack2/8
  MeaModule6/1 -> CAN Pack2/9
  CAN Pack2/1 -> CANPackMessage2/1
  CAN Pack1/1 -> CANPackMessage1/1
  MeaModule9/1 -> WAIT_START/1
  Bus Selector/3 -> BMS_Wo/1  "<BMS_Wo>"
  CAN Pack6/1 -> CANPackMessage6/1
  CAN Pack7/1 -> CANPackMessage7/1
  CANPackMessage6/1 -> CANTransmit6/1
  CANPackMessage7/1 -> CANTransmit7/1
  CANTransmit6/1 -> MeaModule11/1
  CANTransmit7/1 -> MeaModule12/1
  MeaModule11/1 -> Terminator6/1
  MeaModule12/1 -> Terminator7/1
  Bus Selector6/1 -> CAN Pack6/1  "<BatAlmLv>"
  Bus Selector6/2 -> CAN Pack6/2  "<Bat_Current_LSB>"
  Bus Selector6/3 -> CAN Pack6/3  "<Bat_Current_MSB>"
  Bus Selector6/4 -> CAN Pack6/4  "<BatLife>"
  Bus Selector6/5 -> CAN Pack6/5  "<BatSoc>"
  Bus Selector6/6 -> CAN Pack6/6  "<BatSoh>"
  Bus Selector6/7 -> CAN Pack6/7  "<Bat_Voltage_LSB>"
  Bus Selector6/8 -> CAN Pack6/8  "<Bat_Voltage_MSB>"
  Bus Selector7/1 -> CAN Pack7/1  "<BatAlmLv>"
  Bus Selector7/2 -> CAN Pack7/2  "<Bat_Current_LSB>"
  Bus Selector7/3 -> CAN Pack7/3  "<Bat_Current_MSB>"
  Bus Selector7/4 -> CAN Pack7/4  "<BatLife>"
  Bus Selector7/5 -> CAN Pack7/5  "<BatSoc>"
  Bus Selector7/6 -> CAN Pack7/6  "<BatSoh>"
  Bus Selector7/7 -> CAN Pack7/7  "<Bat_Voltage_LSB>"
  Bus Selector7/8 -> CAN Pack7/8  "<Bat_Voltage_MSB>"
  Bus Selector3/1 -> CAN Pack4/1  "<MotControllerTem1>"
  Bus Selector3/2 -> CAN Pack4/2  "<MotControllerem2>"
  Bus Selector3/3 -> CAN Pack4/3  "<Mot_Tem1>"
  Bus Selector3/4 -> CAN Pack4/4  "<Mot_Tem2>"
  Bus Selector3/5 -> MeaModule18/1  "<Re_Mot_SpeedH1>"
  Bus Selector3/6 -> MeaModule17/1  "<Re_Mot_SpeedH2>"
  Bus Selector3/7 -> MeaModule16/1  "<Re_Mot_SpeedL1>"
  Bus Selector3/8 -> MeaModule15/1  "<Re_Mot_SpeedL2>"
  MeaModule14/1 -> CAN Pack3/8
  Bus Selector2/7 -> MeaModule14/1  "<Speed>"
  MeaModule15/1 -> CAN Pack4/8  "Re_Mot_SpeedL2"
  MeaModule16/1 -> CAN Pack4/7  "Re_Mot_SpeedL2"
  MeaModule17/1 -> CAN Pack4/6  "Re_Mot_SpeedL2"
  MeaModule18/1 -> CAN Pack4/5  "Re_Mot_SpeedL2"
  MeaModule19/1 -> CAN Pack5/2  "Re_Mot_SpeedL2"
  Bus Selector2/1 -> CAN Pack3/1  "<Brake>"
  Bus Selector8/1 -> [MODE]  "<MODE>"
  [MODE] -> CAN Pack5/6  "Re_Mot_SpeedL2"
  Bus Selector9/1 -> [H1]  "<DC_BusVoltH1>"
  Bus Selector9/2 -> [L1]  "<DC_BusVoltL1>"
  Bus Selector9/3 -> [H2]  "<DC_BusVoltH2>"
  Bus Selector9/4 -> [L2]  "<DC_BusVoltL2>"
  [H1] -> CAN Pack1/1
  [L1] -> CAN Pack1/2
  [H2] -> CAN Pack2/1
  [L2] -> CAN Pack2/2
  Bus Selector4/1 -> CAN Pack2/4  "<Main_Contactor>"
  Bus Selector1/1 -> CAN Pack1/4  "<Main_Contactor>"

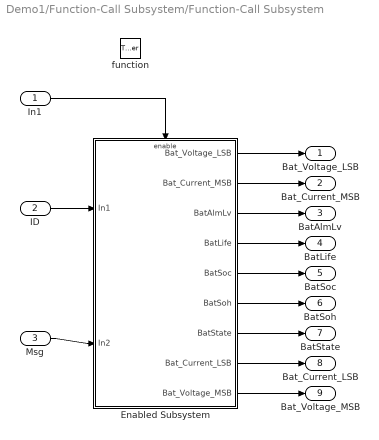
== system Demo1/Function-Call Subsystem/Function-Call Subsystem ==
  In1 : Inport
  ID : Inport  Port=2
  Msg : Inport  Port=3
  function : TriggerPort  TriggerType=function-call  VariantControl=Variant
  Enabled Subsystem : Subsystem  TreatAsAtomicUnit=on
  Bat_Voltage_LSB : Outport
  Bat_Current_MSB : Outport  Port=2
  BatAlmLv : Outport  Port=3
  BatLife : Outport  Port=4
  BatSoc : Outport  Port=5
  BatSoh : Outport  Port=6
  BatState : Outport  Port=7
  Bat_Current_LSB : Outport  Port=8
  Bat_Voltage_MSB : Outport  Port=9
  wires:
  In1/1 -> Enabled Subsystem/Enable
  ID/1 -> Enabled Subsystem/1(In1)
  Msg/1 -> Enabled Subsystem/2(In2)
  Enabled Subsystem/1("Bat_Voltage_LSB ") -> Bat_Voltage_LSB/1
  Enabled Subsystem/2(Bat_Current_MSB) -> Bat_Current_MSB/1
  Enabled Subsystem/3("BatAlmLv ") -> BatAlmLv/1
  Enabled Subsystem/4(BatLife) -> BatLife/1
  Enabled Subsystem/5(BatSoc) -> BatSoc/1
  Enabled Subsystem/6(BatSoh) -> BatSoh/1
  Enabled Subsystem/7(BatState) -> BatState/1
  Enabled Subsystem/8(Bat_Current_LSB) -> Bat_Current_LSB/1
  Enabled Subsystem/9("Bat_Voltage_MSB ") -> Bat_Voltage_MSB/1

== system Demo1/Function-Call Subsystem/Function-Call Subsystem1 ==
  In1 : Inport
  ID : Inport  Port=2
  Msg : Inport  Port=3
  function : TriggerPort  TriggerType=function-call  VariantControl=Variant
  Enabled Subsystem : Subsystem  TreatAsAtomicUnit=on
  Subsystem : Subsystem
  Subsystem1 : Subsystem  Commented=on
  Re_Mot_SpeedH1 : Outport
  Re_Mot_SpeedL1 : Outport  Port=2
  Re_Mot_TorqueH1 : Outport  Port=3
  Re_Mot_TorqueL1 : Outport  Port=4
  MCU1_rdy : Outport  Port=5
  wires:
  Msg/1 -> Enabled Subsystem/2(In2)
  ID/1 -> Enabled Subsystem/1(In1)
  In1/1 -> Enabled Subsystem/Enable
  Enabled Subsystem/1(Pe_Mot_SpeedH1) -> Re_Mot_SpeedH1/1
  Enabled Subsystem/2(Re_MotSpeedL1) -> Re_Mot_SpeedL1/1
  Enabled Subsystem/3(Re_Mot_TorqueH1) -> Re_Mot_TorqueH1/1
  Enabled Subsystem/4(Re_MotTorqueL1) -> Re_Mot_TorqueL1/1
  Enabled Subsystem/5(MCU1State1) -> Subsystem/1(MCU1_State)
  Subsystem/1(MCU1_rdy) -> MCU1_rdy/1

== system Demo1/Function-Call Subsystem/Function-Call Subsystem2 ==
  In1 : Inport
  ID : Inport  Port=2
  Msg : Inport  Port=3
  function : TriggerPort  TriggerType=function-call  VariantControl=Variant
  Enabled Subsystem : Subsystem  TreatAsAtomicUnit=on
  MotControllerTem1 : Outport
  Mot_Tem1 : Outport  Port=2
  DC_BusVoltH1 : Outport  Port=3
  DC_BusVoltL1 : Outport  Port=4
  wires:
  In1/1 -> Enabled Subsystem/Enable
  ID/1 -> Enabled Subsystem/1(In1)
  Msg/1 -> Enabled Subsystem/2(In2)
  Enabled Subsystem/1(MotControllerTem1) -> MotControllerTem1/1
  Enabled Subsystem/2(Mot_Tem1) -> Mot_Tem1/1
  Enabled Subsystem/3(DC_Bus_VoltH1) -> DC_BusVoltH1/1
  Enabled Subsystem/4(DC_Bus_VoltL1) -> DC_BusVoltL1/1

== system Demo1/Function-Call Subsystem/Function-Call Subsystem3 ==
  In1 : Inport
  ID : Inport  Port=2
  Msg : Inport  Port=3
  function : TriggerPort  TriggerType=function-call  VariantControl=Variant
  Enabled Subsystem : Subsystem  TreatAsAtomicUnit=on
  Subsystem : Subsystem
  Re_Mot_SpeedH2 : Outport
  Re_Mot_SpeedL2 : Outport  Port=2
  Re_Mot_TorqueH2 : Outport  Port=3
  Re_Mot_TorqueL2 : Outport  Port=4
  MCU2_rdy : Outport  Port=5
  wires:
  Msg/1 -> Enabled Subsystem/2(In2)
  ID/1 -> Enabled Subsystem/1(In1)
  In1/1 -> Enabled Subsystem/Enable
  Enabled Subsystem/1(Re_Mot_SpeedH2) -> Re_Mot_SpeedH2/1
  Enabled Subsystem/2(Re_Mot_SpeedL2) -> Re_Mot_SpeedL2/1
  Enabled Subsystem/3(Re_Mot_TorqueH2) -> Re_Mot_TorqueH2/1
  Enabled Subsystem/4(Re_Mot_TorqueL2) -> Re_Mot_TorqueL2/1
  Enabled Subsystem/5(MCU2State1) -> Subsystem/1(MCU2_State)
  Subsystem/1(MCU2_rdy) -> MCU2_rdy/1

== system Demo1/Function-Call Subsystem/Function-Call Subsystem4 ==
  In1 : Inport
  ID : Inport  Port=2
  Msg : Inport  Port=3
  function : TriggerPort  TriggerType=function-call  VariantControl=Variant
  Enabled Subsystem : Subsystem  TreatAsAtomicUnit=on
  MotControllerTem2 : Outport
  Mot_Tem2 : Outport  Port=2
  DC_BusVoltH2 : Outport  Port=3
  DC_BusVoltL2 : Outport  Port=4
  wires:
  In1/1 -> Enabled Subsystem/Enable
  ID/1 -> Enabled Subsystem/1(In1)
  Msg/1 -> Enabled Subsystem/2(In2)
  Enabled Subsystem/1(MotControllerTem2) -> MotControllerTem2/1
  Enabled Subsystem/2(Mot_Tem2) -> Mot_Tem2/1
  Enabled Subsystem/4(DC_BusVoltL2) -> DC_BusVoltL2/1
  Enabled Subsystem/3(DC_BusVoltH2) -> DC_BusVoltH2/1

== system Demo1/Function-Call Subsystem/Function-Call Subsystem5 ==
  In1 : Inport
  ID : Inport  Port=2
  Msg : Inport  Port=3
  function : TriggerPort  TriggerType=function-call  VariantControl=Variant
  Enabled Subsystem : Subsystem  TreatAsAtomicUnit=on
  Terminator{,1..4} (5 alike) : Terminator
  MaxTemp : Outport
  wires:
  Msg/1 -> Enabled Subsystem/2(In2)
  ID/1 -> Enabled Subsystem/1(In1)
  In1/1 -> Enabled Subsystem/Enable
  Enabled Subsystem/1("CoolingCtl ") -> Terminator/1
  Enabled Subsystem/2(HeatingCtl) -> Terminator1/1
  Enabled Subsystem/4(MaxTempNo) -> Terminator3/1
  Enabled Subsystem/6(MinTempNo) -> Terminator4/1
  Enabled Subsystem/5(MinTemp) -> Terminator2/1
  Enabled Subsystem/3(MaxTemp) -> MaxTemp/1

== system Demo1/Function-Call Subsystem/Function-Call Subsystem6 ==
  In1 : Inport
  ID : Inport  Port=2
  Msg : Inport  Port=3
  function : TriggerPort  TriggerType=function-call  VariantControl=Variant
  Enabled Subsystem : Subsystem  TreatAsAtomicUnit=on
  Dash_Key : Outport
  wires:
  In1/1 -> Enabled Subsystem/Enable
  ID/1 -> Enabled Subsystem/1(In1)
  Msg/1 -> Enabled Subsystem/2(In2)
  Enabled Subsystem/1(Out1) -> Dash_Key/1

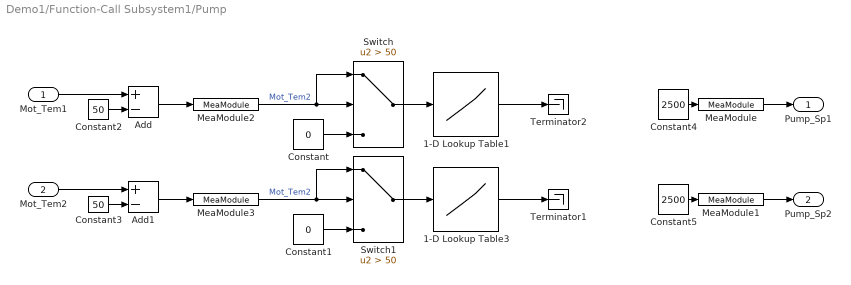
== system Demo1/Function-Call Subsystem1/Pump ==
  Mot_Tem1 : Inport
  Mot_Tem2 : Inport  Port=2
  1-D Lookup Table1 : Lookup_n-D  NumberOfTableDimensions=1  BreakpointsForDimension1=[50 60 70 80 90 100]  BreakpointsForDimension1DataTypeStr=uint16  Table=[0 1000 2000 3000 4000 5000]  TableDataTypeStr=uint16  IntermediateResultsDataTypeStr=uint16  ExtrapMethod=Clip  InternalRulePriority=Speed  OutDataTypeStr=uint16  RndMeth=Simplest  FractionDataTypeStr=double  InputSameDT=on
  1-D Lookup Table3 : Lookup_n-D  NumberOfTableDimensions=1  BreakpointsForDimension1=[50 60 70 80 90 100]  BreakpointsForDimension1DataTypeStr=uint16  Table=PUMP  TableDataTypeStr=uint16  IntermediateResultsDataTypeStr=uint16  ExtrapMethod=Clip  InternalRulePriority=Speed  OutDataTypeStr=uint16  RndMeth=Simplest  FractionDataTypeStr=double  InputSameDT=on
  Add : Sum  Inputs=+-
  Add1 : Sum  Inputs=+-
  Constant : Constant  Value=0  OutDataTypeStr=uint16
  Constant1 : Constant  Value=0  OutDataTypeStr=uint16
  Constant2 : Constant  Value=50
  Constant3 : Constant  Value=50
  Constant4 : Constant  Value=2500  OutDataTypeStr=uint16
  Constant5 : Constant  Value=2500  OutDataTypeStr=uint16
  MeaModule : ec5744lib/RapidECU_U3/07Calibration/MeaModule  signal=PumpL
      settings: SourceProductName=ECUCoder for MPC5744
  MeaModule1 : ec5744lib/RapidECU_U3/07Calibration/MeaModule  signal=PumpR
      settings: SourceProductName=ECUCoder for MPC5744
  MeaModule2 : ec5744lib/RapidECU_U3/07Calibration/MeaModule  signal=Mot_Tem1
      settings: SourceProductName=ECUCoder for MPC5744
  MeaModule3 : ec5744lib/RapidECU_U3/07Calibration/MeaModule  signal=Mot_Tem2
      settings: SourceProductName=ECUCoder for MPC5744
  Switch : Switch  Criteria=u2 > Threshold  Threshold=50
  Switch1 : Switch  Criteria=u2 > Threshold  Threshold=50
  Terminator1 : Terminator
  Terminator2 : Terminator
  Pump_Sp1 : Outport
  Pump_Sp2 : Outport  Port=2
  wires:
  1-D Lookup Table3/1 -> Terminator1/1
  Mot_Tem1/1 -> Add/1
  Mot_Tem2/1 -> Add1/1
  MeaModule2/1 -> Switch/1, Switch/2  "Mot_Tem2"
  Switch/1 -> 1-D Lookup Table1/1
  Constant/1 -> Switch/3
  Constant1/1 -> Switch1/3
  Switch1/1 -> 1-D Lookup Table3/1
  MeaModule3/1 -> Switch1/2, Switch1/1  "Mot_Tem2"
  MeaModule/1 -> Pump_Sp1/1
  MeaModule1/1 -> Pump_Sp2/1
  Add/1 -> MeaModule2/1
  Add1/1 -> MeaModule3/1
  Constant2/1 -> Add/2
  Constant3/1 -> Add1/2
  1-D Lookup Table1/1 -> Terminator2/1
  Constant5/1 -> MeaModule1/1
  Constant4/1 -> MeaModule/1
